simulink model "vib_pro_nim"  (R2016b)
settings: Solver=VariableStepAuto  StartTime=0.0  StopTime=0.1  RelTol=1e-3
settings Model: Creator=diamond  LastModifiedBy=diamond

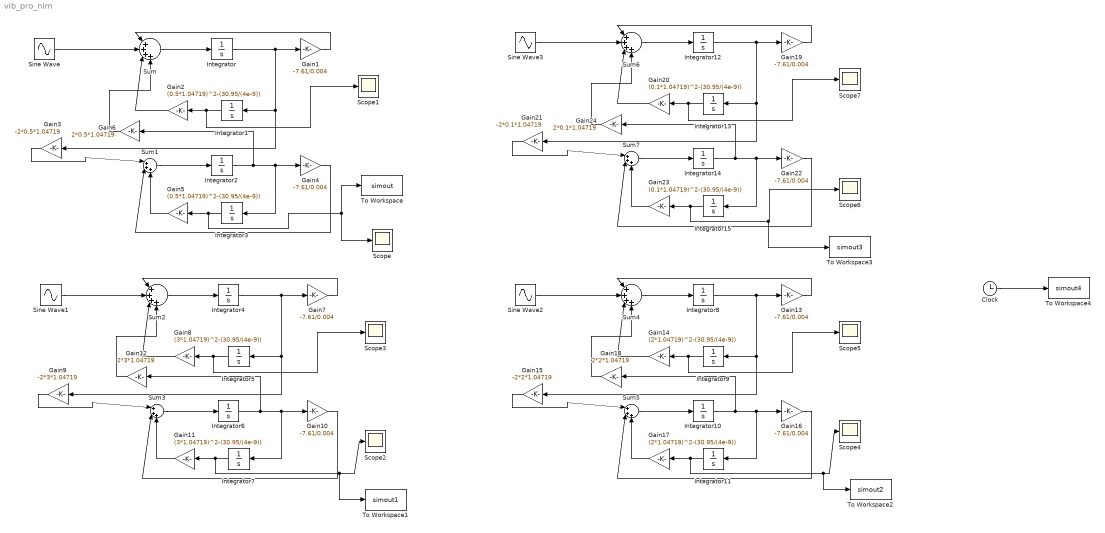
== system vib_pro_nim ==
  Clock : Clock
  Gain{1,4,7,10,13,16,19,22} (8 alike) : Gain  Gain=-7.61/0.004
  Gain11 : Gain  Gain=(3*1.04719)^2-(30.95/(4e-9))
  Gain12 : Gain  Gain=2*3*1.04719
  Gain14 : Gain  Gain=(2*1.04719)^2-(30.95/(4e-9))
  Gain15 : Gain  Gain=-2*2*1.04719
  Gain17 : Gain  Gain=(2*1.04719)^2-(30.95/(4e-9))
  Gain18 : Gain  Gain=2*2*1.04719
  Gain2 : Gain  Gain=(0.5*1.04719)^2-(30.95/(4e-9))
  Gain20 : Gain  Gain=(0.1*1.04719)^2-(30.95/(4e-9))
  Gain21 : Gain  Gain=-2*0.1*1.04719
  Gain23 : Gain  Gain=(0.1*1.04719)^2-(30.95/(4e-9))
  Gain24 : Gain  Gain=2*0.1*1.04719
  Gain3 : Gain  Gain=-2*0.5*1.04719
  Gain5 : Gain  Gain=(0.5*1.04719)^2-(30.95/(4e-9))
  Gain6 : Gain  Gain=2*0.5*1.04719
  Gain8 : Gain  Gain=(3*1.04719)^2-(30.95/(4e-9))
  Gain9 : Gain  Gain=-2*3*1.04719
  Integrator{,2,4,6,8,10,12,14} (8 alike) : Integrator
  Integrator{1,3,5,7,9,11,13,15} (8 alike) : Integrator  InitialCondition=6.39e-6
  Scope{,1..7} (8 alike) : Scope
  Sine Wave{,1..3} (4 alike) : Sin  Amplitude=4.3/0.004  Frequency=2*pi*14e3  SampleTime=0
  Sum{,2,4,6} (4 alike) : Sum  Inputs=|++++
  Sum{1,3,5,7} (4 alike) : Sum  Inputs=|+++
  To Workspace : ToWorkspace  VariableName=simout  SampleTime=-1
  To Workspace1 : ToWorkspace  VariableName=simout1  SampleTime=-1
  To Workspace2 : ToWorkspace  VariableName=simout2  SampleTime=-1
  To Workspace3 : ToWorkspace  VariableName=simout3  SampleTime=-1
  To Workspace4 : ToWorkspace  VariableName=simout4  SampleTime=-1
  wires:
  Clock/1 -> To Workspace4/1
  Sine Wave/1 -> Sum/2
  Sum/1 -> Integrator/1
  Integrator/1 -> Gain1/1, Gain3/1, Integrator1/1
  Integrator1/1 -> Scope1/1, Gain2/1
  Gain2/1 -> Sum/3
  Sum1/1 -> Integrator2/1
  Integrator2/1 -> Integrator3/1, Gain4/1, Gain6/1
  Gain4/1 -> Sum1/2
  Integrator3/1 -> To Workspace/1, Scope/1, Gain5/1
  Gain5/1 -> Sum1/3
  Gain3/1 -> Sum1/1
  Gain6/1 -> Sum/4
  Gain1/1 -> Sum/1
  Sine Wave1/1 -> Sum2/2
  Sum2/1 -> Integrator4/1
  Integrator4/1 -> Gain7/1, Gain9/1, Integrator5/1
  Integrator5/1 -> Scope3/1, Gain8/1
  Gain8/1 -> Sum2/3
  Sum3/1 -> Integrator6/1
  Integrator6/1 -> Integrator7/1, Gain10/1, Gain12/1
  Gain10/1 -> Sum3/2
  Integrator7/1 -> To Workspace1/1, Scope2/1, Gain11/1
  Gain11/1 -> Sum3/3
  Gain9/1 -> Sum3/1
  Gain12/1 -> Sum2/4
  Gain7/1 -> Sum2/1
  Sine Wave3/1 -> Sum6/2
  Sum6/1 -> Integrator12/1
  Integrator12/1 -> Gain19/1, Gain21/1, Integrator13/1
  Integrator13/1 -> Scope7/1, Gain20/1
  Gain20/1 -> Sum6/3
  Sum7/1 -> Integrator14/1
  Integrator14/1 -> Integrator15/1, Gain22/1, Gain24/1
  Gain22/1 -> Sum7/2
  Integrator15/1 -> To Workspace3/1, Scope6/1, Gain23/1
  Gain23/1 -> Sum7/3
  Gain21/1 -> Sum7/1
  Gain24/1 -> Sum6/4
  Gain19/1 -> Sum6/1
  Sine Wave2/1 -> Sum4/2
  Sum4/1 -> Integrator8/1
  Integrator8/1 -> Gain13/1, Gain15/1, Integrator9/1
  Integrator9/1 -> Scope5/1, Gain14/1
  Gain14/1 -> Sum4/3
  Sum5/1 -> Integrator10/1
  Integrator10/1 -> Integrator11/1, Gain16/1, Gain18/1
  Gain16/1 -> Sum5/2
  Integrator11/1 -> To Workspace2/1, Scope4/1, Gain17/1
  Gain17/1 -> Sum5/3
  Gain15/1 -> Sum5/1
  Gain18/1 -> Sum4/4
  Gain13/1 -> Sum4/1
